simulink model "SiDynoReferenceApplication"  (R2020a)
settings: Solver=ode23tb  StartTime=0.0  StopTime=15000  RelTol=1e-3  EnableMultiTasking=on
model workspace (MAT data in the model file):
  DynOperatingPts = timeseries
  DynOperatingPts.Name = 'Dynamic Operating Points'
  DynOperatingPts.DataInfo = tsdata.datametadata
  DynOperatingPts.DataInfo.Interpolation = tsdata.interpolation
  DynOperatingPts.DataInfo.Interpolation.Fhandle : function handle (value not decoded)
  DynOperatingPts.DataInfo.Interpolation.Name = 'linear'
  DynOperatingPts.TimeInfo = tsdata.timemetadata
  DynOperatingPts.TimeInfo.Length = 1281
  DynOperatingPts.TimeInfo.DuplicateTimes = 0
  DynOperatingPts.TimeInfo.Time_ = [0 0.001 7.75860549558 7.75960549558 8.75958684985 8.76058684985 10.7615495584 10.7625495584 11.7625309127 11.7635309127 13.7644936212 13.7654936212 ... (1281 elements, 1281x1)]
  DynOperatingPts.TimeInfo.Initialized = 1
  DynOperatingPts.QualityInfo = tsdata.qualmetadata
  DynOperatingPts.Data_ = [0 750 750 750 750 750 750 750 750 750 750 750 ... (2562 elements, 1281x2)]
  MaxTurboSpd = 232000
  SteadyEngSpdCmdPts = [750 750 750 750 750 750 750 750 750 750 750 750 ... (225 elements, 15x15)]
  SteadyStateWaitLimit = 100
  SteadyTrqCmdPts = [15 30.3571428571 45.7142857143 61.0714285714 76.4285714286 91.7857142857 107.142857143 122.5 137.857142857 153.214285714 168.571428571 183.928571429 ... (225 elements, 15x15)]
undefined symbols (not defined in the file or in its folder): DynoResultsBlock, GenerateMappedEngineCalibrations, InjPw, RecalibrateSIController, ThrPosPctCmd, WgAreaPctCmd
libraries: autolibutils x2, simulink x2, autolibpowerinfoutils x1
(part 1 of 2)
settings Model: ModifiedByFormat=The MathWorks, Inc.  SimulationMode=accelerator  PauseTimes=4395  NumberOfSteps=1000  SnapshotBufferSize=20  SnapshotInterval=1000  OrderedModelArguments=off  Creator=The MathWorks, Inc.  LastModifiedBy=The MathWorks, Inc.
settings SolverCC: DecoupledContinuousIntegration=on  MinimalZcImpactIntegration=on
settings DataIOCC: SaveOutput=off  SignalLogging=off  DSMLogging=off  SaveTime=off  ReturnWorkspaceOutputs=off
settings OptimizationCC: SimCompilerOptimization=on
settings DebuggingCC: UnderspecifiedInitializationDetection=Classic  MergeDetectMultiDrivingBlocksExec=none  PregeneratedLibrarySubsystemCodeDiagnostic=none  ArithmeticOperatorsInVariantConditions=warning
settings ModelReferenceCC: UpdateModelReferenceTargets=IfOutOfDate  ModelReferenceMinAlgLoopOccurrences=on  PropagateSignalLabelsOutOfModel=off
settings SFSimCC: SimUseLocalCustomCode=off
settings RTWCC: RTWUseLocalCustomCode=off  BuildConfiguration=Faster Runs  RTWCompilerOptimization=on
settings CodeAppCC: StateflowObjectComments=on
settings GRTTargetCC: TargetLangStandard=C89/C90 (ANSI)
settings ConfigComp: CovMetricSettings=dsw  CovHtmlReporting=on  CovSaveCumulativeToWorkspaceVar=on  CovSaveSingleToWorkspaceVar=on  CovShowResultsExplorer=off  CovExternalEMLEnable=off

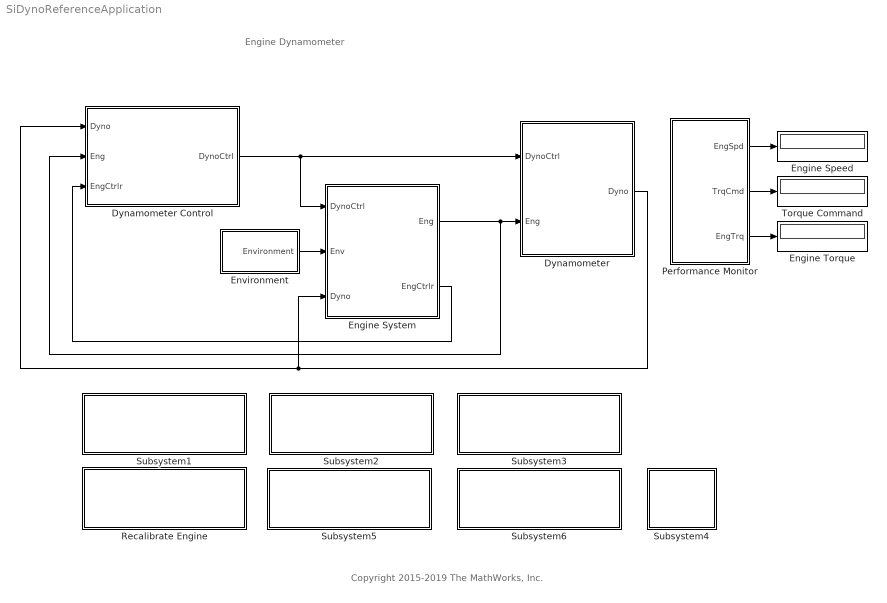
== system SiDynoReferenceApplication ==
  note: Engine Dynamometer
  note: Copyright 2015-2019 The MathWorks, Inc.
  Dynamometer : Subsystem
  Dynamometer Control : Subsystem  Variant=on  VariantControlMode=Label  LabelModeActiveChoice=CalThrWg
  Engine Speed : Display
      settings: Decimation=100
  Engine System : Subsystem
      mask Display:
      | TaggedBlk = find_system(gcb, 'LookUnderMasks', 'All', 'Tag', 'MappedEngCalByMBC');
      | ImageName = which('mbc_app_24.png');
      | 
      | if ~isempty(TaggedBlk)
      |     if ~isempty(ImageName)
      |         IconImg = imread(ImageName,'png');
      |         MaskImg = 256*ones(150, 150,3);
      |         MaskImg = uint8(MaskImg);
      |         Xstart = 125;
      |         Ystart = 0;
      |         MaskImg((1:size(IconImg, 1))+Ystart, (1:size(IconImg, 2))+Xstart, 1:3) = IconImg;
      |         image(MaskImg);
      |     end
      |     disp('Mapped Engine\n Calibrated by\nMBC Toolbox')
      | end
  Engine Torque : Display
      settings: Decimation=100
  Environment : Subsystem
  Performance Monitor : Subsystem  StartFcn=DynoResultsBlock(gcb, 'StartFcn');  StopFcn=DynoResultsBlock(gcb, 'StopFcn');  mask(Performance Monitor){SteadyWsVarName=SteadyDynoSimOut, XVarPopup=Engine speed (rpm), YVarPopup=Torque command (N*m), ZVarPopup=Measured engine torque (N*m), DynWsVarName=DynamicDynoSimOut, DispAtEndCheckbox=on, UseSdiViewCheckbox=on, SdiRunName=Dynamometer Results, SdiViewFileName=DynoSDI_config.mldatx, ShowWaitbarCheckbox=on}
      mask prompts: SteadyWsVarName "Steady state "To Workspace" variable name:"; XVarPopup "X axis variable:"; YVarPopup "Y axis variable:"; ZVarPopup "Z axis variable:"; DynWsVarName "Dynamic "To Workspace" variable name:"; DispAtEndCheckbox "Display results at end of simulation"; UseSdiViewCheckbox "Open Simulation Data Inspector view"; SdiRunName "Simulation Data Inspector run name:"; SdiViewFileName "Simulation Data Inspector view file name:"; ShowWaitbarCheckbox "Show wait bar"
      mask init:
      | DynoResultsBlock(gcb, 'Initialization');
      mask Help: helpview([docroot,'/toolbox/autoblks/helptargets.map'], 'siengine_dyno_refapp')
      mask TypeOptions XVarPopup: Air-fuel ratio | BSFC (g/(kW*hr)) | Compressor outlet temperature (C) | Compressor pressure ratio | EGR cooler outlet temperature (C) | EGR mass flow rate (g/s) | EGR percent | EGR valve area percent | EGR valve area percent command | Engine speed (rpm) | Engine speed command (rpm) | Estimated intake port mass flow rate (g/s) | Exhaust cam phase (degCrkRet) | Exhaust cam phase command (degCrkRet) | Exhaust manifold temperature (C) | Fuel mass flow rate (g/s) | Idle speed control torque command (N*m) | Injection pulse width (ms) | Intake cam phase (degCrkAdv) | Intake cam phase command (degCrkAdv) | Intake manifold pressure (kPa) | Intake manifold temperature (C) | Intake port mass flow rate (g/s) | Intercooler outlet temperature (C) | Load command | Measured engine torque (N*m) | Normalized air charge | Percent complete | Spark advance (degCrkAdv) | Steady state flag | Tailpipe CO emissions (g/s) | Tailpipe CO2 emissions (g/s) | Tailpipe HC emissions (g/s) | Tailpipe NOx emissions (g/s) | Throttle position percent | Throttle position percent command | Time (s) | Torque command (N*m) | Turbine outlet temperature (C) | Turbine pressure ratio | Turbocharger rack position | Turbocharger rack position command | Turbocharger shaft speed (rpm) | Wastegate area percent | Wastegate area percent command
      mask TypeOptions YVarPopup: None | Air-fuel ratio | BSFC (g/(kW*hr)) | Compressor outlet temperature (C) | Compressor pressure ratio | EGR cooler outlet temperature (C) | EGR mass flow rate (g/s) | EGR percent | EGR valve area percent | EGR valve area percent command | Engine speed (rpm) | Engine speed command (rpm) | Estimated intake port mass flow rate (g/s) | Exhaust cam phase (degCrkRet) | Exhaust cam phase command (degCrkRet) | Exhaust manifold temperature (C) | Fuel mass flow rate (g/s) | Idle speed control torque command (N*m) | Injection pulse width (ms) | Intake cam phase (degCrkAdv) | Intake cam phase command (degCrkAdv) | Intake manifold pressure (kPa) | Intake manifold temperature (C) | Intake port mass flow rate (g/s) | Intercooler outlet temperature (C) | Load command | Measured engine torque (N*m) | Normalized air charge | Percent complete | Spark advance (degCrkAdv) | Steady state flag | Tailpipe CO emissions (g/s) | Tailpipe CO2 emissions (g/s) | Tailpipe HC emissions (g/s) | Tailpipe NOx emissions (g/s) | Throttle position percent | Throttle position percent command | Time (s) | Torque command (N*m) | Turbine outlet temperature (C) | Turbine pressure ratio | Turbocharger rack position | Turbocharger rack position command | Turbocharger shaft speed (rpm) | Wastegate area percent | Wastegate area percent command
      mask TypeOptions ZVarPopup: None | Air-fuel ratio | BSFC (g/(kW*hr)) | Compressor outlet temperature (C) | Compressor pressure ratio | EGR cooler outlet temperature (C) | EGR mass flow rate (g/s) | EGR percent | EGR valve area percent | EGR valve area percent command | Engine speed (rpm) | Engine speed command (rpm) | Estimated intake port mass flow rate (g/s) | Exhaust cam phase (degCrkRet) | Exhaust cam phase command (degCrkRet) | Exhaust manifold temperature (C) | Fuel mass flow rate (g/s) | Idle speed control torque command (N*m) | Injection pulse width (ms) | Intake cam phase (degCrkAdv) | Intake cam phase command (degCrkAdv) | Intake manifold pressure (kPa) | Intake manifold temperature (C) | Intake port mass flow rate (g/s) | Intercooler outlet temperature (C) | Load command | Measured engine torque (N*m) | Normalized air charge | Percent complete | Spark advance (degCrkAdv) | Steady state flag | Tailpipe CO emissions (g/s) | Tailpipe CO2 emissions (g/s) | Tailpipe HC emissions (g/s) | Tailpipe NOx emissions (g/s) | Throttle position percent | Throttle position percent command | Time (s) | Torque command (N*m) | Turbine outlet temperature (C) | Turbine pressure ratio | Turbocharger rack position | Turbocharger rack position command | Turbocharger shaft speed (rpm) | Wastegate area percent | Wastegate area percent command
      mask DialogControl SteadyStateGroup Prompt: Steady state
      mask DialogControl SteadyDesc Prompt: Plot steady-state simulation results. Data is logged when an operating point reaches steady state. Once all operating points simulate, the dynamometer outputs data to base workspace. Plot the logged data as a function of 1 or 2 variables. Specify 'None' for the Z axis variable to create a 2D plot. Specify X, Y, and Z variable names to create a surface plot.
      mask DialogControl PlotSteadyButton Prompt: Plot Steady State Results
      mask DialogControl PlotSteadyButton Callback: DynoResultsBlock(gcb, 'PlotSteadyButtonCallback');
      mask DialogControl DynamicGroup Prompt: Dynamic
      mask DialogControl DynamicDesc Prompt: Plot dynamic results using Simulation Data Inspector.
      mask DialogControl PlotDynamicButton Prompt: Plot Dynamic Results
      mask DialogControl PlotDynamicButton Callback: DynoResultsBlock(gcb, 'PlotDynamicButtonCallback');
      mask DialogControl WaitbarGroup Prompt: Wait bar
  Recalibrate Engine : Subsystem  mask{EngReszSpecType=Power, EngReszMaxPwrDesIn=115.0917, EngReszDispDesIn=1.5, EngReszMaxPwrDes=115.0917, EngReszNumCylDes=4, EngReszMaxPwr=115.0917, EngReszNumCyl=4, EngReszDisp=1.5, EngReszIdleSpd=750, EngReszMaxTqSpd=2571, EngReszMaxTq=230.6, EngReszBestFuelPwr=41.1, EngReszBestFuelSpd=2571, EngReszBestFuelTq=152.7, EngReszBestFuelBSFC=225.9, EngReszSpdMaxPwr=5000, EngReszTqMaxPwr=219.8, EngReszThrDiam=50, EngReszIntkManVol=2.86, EngReszExhManVol=1.6, EngReszCompOutVol=2.6, EngReszMaxTurboSpd=232000, EngReszTurboRotInert=0.016, EngReszInjSlp=6.45}
      mask prompts: EngReszSpecType "Power or displacement"; EngReszMaxPwrDesIn "Desired maximum power [kW]:"; EngReszDispDesIn "Desired displacement [L]:"; EngReszMaxPwrDes "Desired maximum power [kW]:"; EngReszNumCylDes "Desired number of cylinders:"; EngReszMaxPwr "Maximum power [kW]:"; EngReszNumCyl "Number of cylinders:"; EngReszDisp "Engine displacement [L]:"; EngReszIdleSpd "Idle speed [rpm]:"; EngReszMaxTqSpd "Speed for maximum torque [rpm]:"; EngReszMaxTq "Maximum torque [Nm]:"; EngReszBestFuelPwr "Power for best fuel [kW]:"; EngReszBestFuelSpd "Speed for best fuel [rpm]:"; EngReszBestFuelTq "Torque for best fuel [Nm]:"; EngReszBestFuelBSFC "BSFC for best fuel [g/kWh]:"; EngReszSpdMaxPwr "Speed for maximum power [rpm]:"; EngReszTqMaxPwr "Torque for maximum power [Nm]:"; EngReszThrDiam "Throttle bore diameter [mm]:"; EngReszIntkManVol "Intake manifold volume [L]:"; EngReszExhManVol "Exhaust manifold volume [L]:"; EngReszCompOutVol "Compressor out volume [L]:"; EngReszMaxTurboSpd "Maximum turbo speed [rpm]:"; EngReszTurboRotInert "Turbo rotor inertia [kg*m^2]:"; EngReszInjSlp "Fuel injector slope [mg/ms]:"
      mask help: Resize engine plant and re-calibrate engine controller based on desired maximum power level or displacement, and number of cylinders
      settings: OpenFcn=|
      | block=[bdroot '/Recalibrate Engine'];
      | 
      | modelStatus = get_param(bdroot,'SimulationStatus');
      | 
      | if ~bdIsLibrary(bdroot) && strcmp(modelStatus,'stopped')
      |    autoicon('autolibsiengresize',block,'open');
      |    open_system(block,'mask');
      | elseif ~bdIsLibrary(bdroot) && ~strcmp(modelStatus,'stopped')
      | else
      | end
      | 
      | clear modelStatus;
      | clear block;
      mask Help: eval('autoblkshelp(''pt_si_resize'')');
      mask TypeOptions EngReszSpecType: Power | Displacement
      mask Callback EngReszSpecType: autoicon('autolibsiengresize',gcb,'resizebasis');
      mask DialogControl DescGroupVar Prompt: Engine resize and recalibrate tool
      mask DialogControl DescTextVar Prompt: Resize engine plant and re-calibrate engine controller based on desired maximum power level or displacement, and number of cylinders
      mask DialogControl ResizeEngButton Prompt: Resize Engine
      mask DialogControl ResizeEngButton Callback: autoicon('autolibsiengresize',gcb,'resize');
      mask DialogControl CurrEngDesign Prompt: Current Engine Design
      mask Display: disp('Resize Engine and\nRecalibrate Controller')
  Subsystem1 : Subsystem
      settings: OpenFcn=DynamometerStart(gcb, 'SteadyState')
      mask Display: disp('Execute Engine Mapping\nExperiment')
  Subsystem2 : Subsystem
      settings: OpenFcn=DynamometerStart(gcb, 'Dynamic')
      mask Display: disp('Execute Model Predictive\nControl Plant Model Experiment')
  Subsystem3 : Subsystem  StopFcn=RecalibrateSIController(gcb, 'StopFcn')
      settings: OpenFcn=RecalibrateSIController(gcb, 'OpenFcn')
      mask Display: disp('Recalibrate Controller')
  Subsystem4 : Subsystem
      settings: OpenFcn=helpview([docroot,'/toolbox/autoblks/helptargets.map'], 'siengine_dyno_refapp')
      mask Display: disp('Help')
  Subsystem5 : Subsystem  LoadFcn=GenerateMappedEngineCalibrations(gcb, 'CheckMBCLicense');  mask(Create Mapped Engine from Spreadsheet){SpreadsheetFileName=SiEngineData.xlsx, MBCProjectName=EngDataMBCProject.mat, CageFileName=MappedEngCageTbls.cag, MappedEngMdlRefName=SiMappedEngine}
      mask prompts: SpreadsheetFileName "Spreadsheet file:"; MBCProjectName "MBC project name:"; CageFileName "CAGE file name:"; MappedEngMdlRefName "Mapped engine model reference name"
      mask help: Use Model-Based Calibration Toolbox to generate a mapped engine calibration from a data spreadsheet. Apply the calibration to a Powertrain Blockset mapped engine model.
      mask init:
      | GenerateMappedEngineCalibrations(gcb, 'Init');
      settings: OpenFcn=open_system(gcb, 'mask')
      mask Help: helpview([docroot,'/toolbox/autoblks/helptargets.map'], 'siengine_dyno_spreadsheet')
      mask DialogControl MBCHyperlink Prompt: Requires Model-Based Calibration Toolbox
      mask DialogControl MBCHyperlink Callback: helpview([docroot,'/toolbox/autoblks/helptargets.map'], 'siengine_dyno_refapp')
      mask DialogControl Container3 Prompt: Step 1: Generate mapped engine calibration using Model-Based Calibration Toolbox
      mask DialogControl SpreadsheetFileNameSelect Prompt: ...
      mask DialogControl SpreadsheetFileNameSelect Callback: GenerateMappedEngineCalibrations(gcb, 'SpreadsheetFileNameSelect');
      mask DialogControl GenMappedEngCalButton Prompt: Generate mapped engine calibration
      mask DialogControl GenMappedEngCalButton Callback: GenerateMappedEngineCalibrations(gcb, 'GenMappedEngCalButton');
      mask DialogControl Container4 Prompt: Step 2: Apply calibration to mapped engine model
      mask DialogControl ApplyCalMappedEngButton Prompt: Apply calibration to mapped engine model
      mask DialogControl ApplyCalMappedEngButton Callback: GenerateMappedEngineCalibrations(gcb, 'ApplyCalMappedEngButton');
      mask Display: disp('Generate Mapped Engine\nfrom Spreadsheet')
  Subsystem6 : Subsystem  mask(Create Mapped Engine from Spreadsheet){SpreadsheetFileName=SiEngineData.xlsx, MBCProjectName=EngDataMBCProject.mat, CageFileName=MappedEngCageTbls.cag, MappedEngMdlRefName=SiMappedEngine}
      mask prompts: SpreadsheetFileName "Spreadsheet file:"; MBCProjectName "MBC project name:"; CageFileName "CAGE file name:"; MappedEngMdlRefName "Mapped engine model reference name"
      mask help: Use Model-Based Calibration Toolbox to generate a mapped engine calibration from a data spreadsheet. Apply the calibration to a Powertrain Blockset mapped engine model.
      mask init:
      | GenerateMappedEngineCalibrations(gcb, 'Init');
      settings: OpenFcn=[~,~,~,~,~,~,~,~,~,~,~,~,~,~]=FitSiEngineLSTM(bdroot(gcb));
      mask Help: helpview([docroot,'/toolbox/autoblks/helptargets.map'], 'siengine_dyno_spreadsheet')
      mask DialogControl MBCHyperlink Prompt: Requires Model-Based Calibration Toolbox
      mask DialogControl MBCHyperlink Callback: helpview([docroot,'/toolbox/autoblks/helptargets.map'], 'siengine_dyno_refapp')
      mask DialogControl Container3 Prompt: Step 1: Generate mapped engine calibration using Model-Based Calibration Toolbox
      mask DialogControl SpreadsheetFileNameSelect Prompt: ...
      mask DialogControl SpreadsheetFileNameSelect Callback: GenerateMappedEngineCalibrations(gcb, 'SpreadsheetFileNameSelect');
      mask DialogControl GenMappedEngCalButton Prompt: Generate mapped engine calibration
      mask DialogControl GenMappedEngCalButton Callback: GenerateMappedEngineCalibrations(gcb, 'GenMappedEngCalButton');
      mask DialogControl Container4 Prompt: Step 2: Apply calibration to mapped engine model
      mask DialogControl ApplyCalMappedEngButton Prompt: Apply calibration to mapped engine model
      mask DialogControl ApplyCalMappedEngButton Callback: GenerateMappedEngineCalibrations(gcb, 'ApplyCalMappedEngButton');
      mask Display: disp('Generate Deep Learning\nEngine Model ')
  Torque Command : Display
      settings: Decimation=100
  wires:
  Performance Monitor/3(EngTrq) -> Engine Torque/1
  Performance Monitor/2(TrqCmd) -> Torque Command/1
  Performance Monitor/1(EngSpd) -> Engine Speed/1
  Engine System/2(EngCtrlr) -> Dynamometer Control/3(EngCtrlr)
  Dynamometer Control/1(DynoCtrl) -> Dynamometer/1(DynoCtrl), Engine System/1(DynoCtrl)
  Dynamometer/1(Dyno) -> Dynamometer Control/1(Dyno), Engine System/3(Dyno)
  Engine System/1(Eng) -> Dynamometer Control/2(Eng), Dynamometer/2(Eng)
  Environment/1(Environment) -> Engine System/2(Env)

== system SiDynoReferenceApplication/Dynamometer ==
  DynoCtrl : Inport
  Eng : Inport  Port=2
  Bus Creator : BusCreator  Inputs=2
  Bus Selector : BusSelector  OutputSignals=EngPlnt.EngTrq,EngPlnt.EngSpd
  Dynamometer Motor Controller : Subsystem
  Dynamometer Plant : Subsystem
  Dyno : Outport  VectorParamsAs1DForOutWhenUnconnected=off
  tag scope: DynoResults=global
  wires:
  Bus Creator/1 -> Dyno/1, [DynoResults]
  Eng/1 -> Bus Selector/1, Dynamometer Plant/1(Eng), Dynamometer Motor Controller/1(EngPlnt)
  Dynamometer Plant/1(DynoPlnt) -> [DynoPlnt], Dynamometer Motor Controller/3(DynoPlnt)
  Dynamometer Motor Controller/1(DynoMotorCtrl) -> Dynamometer Plant/4(DynoCtrl)
  [DynoPlnt] -> Bus Creator/2  "DynoPlnt"
  [DynoCtrl] -> Bus Creator/1  "DynoCtrl"
  DynoCtrl/1 -> [DynoCtrl], Dynamometer Motor Controller/2(DynoCtrl)
  Bus Selector/1 -> Dynamometer Plant/2(EngTrq)  "<EngTrq>"
  Bus Selector/2 -> Dynamometer Plant/3("EngSpd ")  "<EngSpd>"

== system SiDynoReferenceApplication/Dynamometer Control ==
  Dyno : Inport
  Eng : Inport  Port=2
  EngCtrlr : Inport  Port=3
  Calibrate Throttle and Wastegate : Subsystem  VariantControl=CalThrWg
  Dynamic : Subsystem  VariantControl=Dynamic
  Steady State : Subsystem  VariantControl=SteadyState
  DynoCtrl : Outport  VectorParamsAs1DForOutWhenUnconnected=off

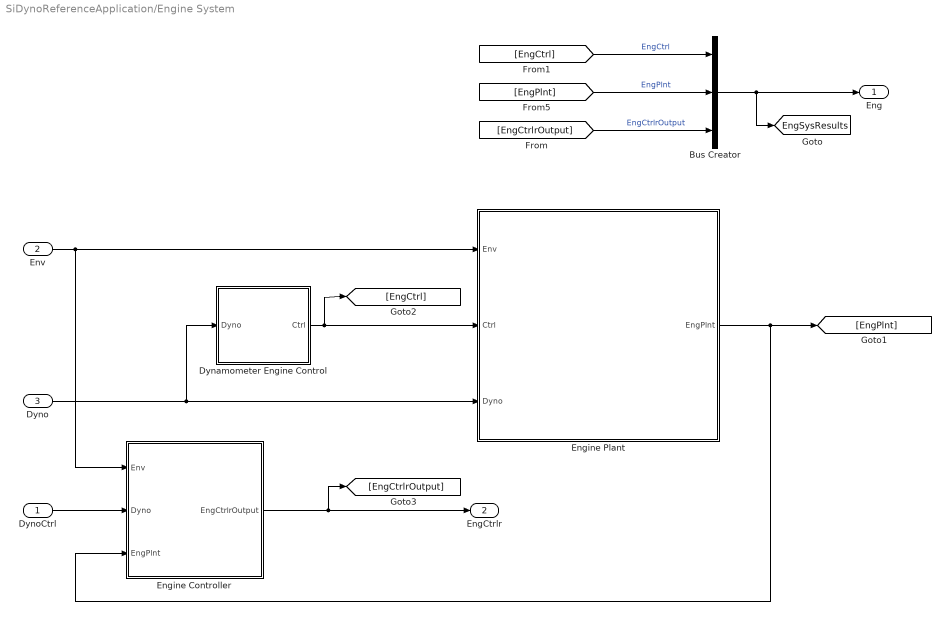
== system SiDynoReferenceApplication/Engine System ==
  DynoCtrl : Inport
  Env : Inport  Port=2
  Dyno : Inport  Port=3
  Bus Creator : BusCreator  Inputs=3
  Dynamometer Engine Control : Subsystem
  Engine Controller : Subsystem
  Engine Plant : Subsystem
  Eng : Outport  VectorParamsAs1DForOutWhenUnconnected=off
  EngCtrlr : Outport  Port=2  VectorParamsAs1DForOutWhenUnconnected=off
  tag scope: EngSysResults=global
  wires:
  Dynamometer Engine Control/1(Ctrl) -> Engine Plant/2(Ctrl), [EngCtrl]
  Dyno/1 -> Dynamometer Engine Control/1(Dyno), Engine Plant/3(Dyno)
  Env/1 -> Engine Controller/1(Env), Engine Plant/1(Env)
  Engine Plant/1(EngPlnt) -> [EngPlnt], Engine Controller/3(EngPlnt)
  Bus Creator/1 -> Eng/1, [EngSysResults]
  [EngPlnt] -> Bus Creator/2  "EngPlnt"
  [EngCtrl] -> Bus Creator/1  "EngCtrl"
  Engine Controller/1(EngCtrlrOutput) -> EngCtrlr/1, [EngCtrlrOutput]
  [EngCtrlrOutput] -> Bus Creator/3  "EngCtrlrOutput"
  DynoCtrl/1 -> Engine Controller/2(Dyno)

== system SiDynoReferenceApplication/Environment ==
  Bus Creator : BusCreator  Inputs=4
  Bus Creator3 : BusCreator  Inputs=3
  Bus Creator4 : BusCreator  Inputs=2
  Bus Creator5 : BusCreator  Inputs=2
  Constant : Constant  Value=1.*ones(4,1)
  Constant1 : Constant  Value=1.*ones(4,1)
  Constant{2..5} (4 alike) : Constant  Value=0
  Constant6 : Constant  Value=300
  Constant7 : Constant  Value=101325
  Environment : Outport  VectorParamsAs1DForOutWhenUnconnected=off
  wires:
  Constant/1 -> Bus Creator5/1  "lam_mu_x"
  Constant1/1 -> Bus Creator5/2  "lam_mu_y"
  Bus Creator5/1 -> Bus Creator4/2  "Ground_mu"
  Bus Creator4/1 -> Bus Creator/3  "Ground"
  Bus Creator3/1 -> Bus Creator/4  "Wind"
  Constant3/1 -> Bus Creator3/1  "wind_x"
  Constant4/1 -> Bus Creator3/2  "wind_y"
  Constant5/1 -> Bus Creator3/3  "wind_z"
  Constant6/1 -> Bus Creator/1  "Temp"
  Constant2/1 -> Bus Creator4/1  "Grade"
  Bus Creator/1 -> Environment/1  "Environment"
  Constant7/1 -> Bus Creator/2  "Baro"

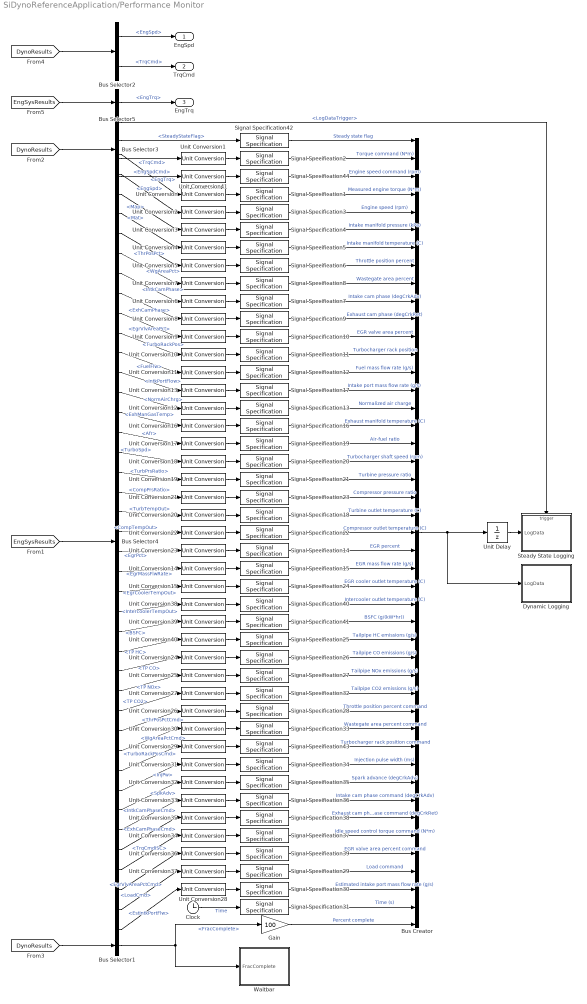
== system SiDynoReferenceApplication/Performance Monitor ==
  Bus Creator : BusCreator  Inputs=45
  Bus Selector1 : BusSelector  OutputSignals=DynoCtrl.DynoCtrl.FracComplete
  Bus Selector2 : BusSelector  OutputSignals=DynoPlnt.EngSpd,DynoCtrl.DynoCtrl.TrqCmd
  Bus Selector3 : BusSelector  OutputSignals=DynoCtrl.DynoCtrl.LogDataTrigger,DynoCtrl.DynoCtrl.SteadyStateFlag,DynoCtrl.DynoCtrl.TrqCmd,DynoCtrl.DynoCtrl.EngSpdCmd
  Bus Selector4 : BusSelector  OutputSignals=EngPlnt.EngTrq,EngPlnt.EngSpd,EngPlnt.Map,EngPlnt.Mat,EngPlnt.ThrPosPct,EngPlnt.WgAreaPct,EngPlnt.IntkCamPhase,EngPlnt.ExhCamPhase,EngPlnt.EgrVlvAreaPct,EngPlnt.TurboRackPos,EngPlnt.FuelFlw,EngPlnt.IntkPortFlow,EngPlnt.NormAirChrg,EngPlnt.ExhManGasTemp,EngPlnt.Afr,EngPlnt.TurboSpd,EngPlnt.TurbPrsRatio,EngPlnt.CompPrsRatio,EngPlnt.TurbTempOut,EngPlnt.CompTempOut,EngPlnt.EgrPct,EngPlnt.EgrMassFlwRate,EngPlnt.EgrCoolerTempOut,EngPlnt.IntercoolerTempOut,EngPlnt.BSFC,EngPlnt.TP HC,EngPlnt.TP CO,EngPlnt.TP NOx,EngPlnt.TP CO2,EngCtrl.ThrPosPctCmd,EngCtrl.WgAreaPctCmd,EngCtrl.TurboRackPosCmd,EngCtrl.InjPw,EngCtrl.SpkAdv,EngCtrl.IntkCamPhaseCmd,EngCtrl.ExhCamPhaseCmd,EngCtrl.TrqCmdISC,EngCtrl.EgrVlvAreaPctCmd,EngCtrl.LoadCmd,EngCtrl.EstIntkPortFlw
  Bus Selector5 : BusSelector  OutputSignals=EngPlnt.EngTrq
  Clock : Clock
  Dynamic Logging : Subsystem
  Gain : Gain  Gain=100
  Signal Specification1 : SignalSpecification  Unit=N*m
  Signal Specification{6,8,10,14,28,33,39} (7 alike) : SignalSpecification  Unit=%
  Signal Specification{11,13,19,21,23,29,42..43} (8 alike) : SignalSpecification  Unit=1
  Signal Specification{12,15,17,25..27,30,32} (8 alike) : SignalSpecification  Unit=g/s
  Signal Specification{5,16,18,22,24,40} (6 alike) : SignalSpecification  Unit=°C
  Signal Specification2 : SignalSpecification  Unit=N*m
  Signal Specification20 : SignalSpecification  Unit=rpm
  Signal Specification3 : SignalSpecification  Unit=rpm
  Signal Specification31 : SignalSpecification  Unit=s
  Signal Specification34 : SignalSpecification  Unit=ms
  Signal Specification{7,9,35..36,38} (5 alike) : SignalSpecification  Unit=deg
  Signal Specification37 : SignalSpecification  Unit=N*m
  Signal Specification4 : SignalSpecification  Unit=kPa
  Signal Specification41 : SignalSpecification  Unit=g/(kW*hr)
  Signal Specification44 : SignalSpecification  Unit=rpm
  Steady State Logging : Subsystem
  Unit Conversion{,1..41} (42 alike) : UnitConversion
  Unit Delay : UnitDelay  SampleTime=-1  HasFrameUpgradeWarning=on
  Waitbar : Subsystem  StartFcn=""
  EngSpd : Outport  VectorParamsAs1DForOutWhenUnconnected=off
  TrqCmd : Outport  Port=2  VectorParamsAs1DForOutWhenUnconnected=off
  EngTrq : Outport  Port=3  VectorParamsAs1DForOutWhenUnconnected=off
  wires:
  Gain/1 -> Bus Creator/45  "Percent complete"
  Signal Specification9/1 -> Bus Creator/11  "Exhaust cam phase (degCrkRet)"
  Signal Specification8/1 -> Bus Creator/9  "Wastegate area percent"
  Signal Specification7/1 -> Bus Creator/10  "Intake cam phase (degCrkAdv)"
  Signal Specification6/1 -> Bus Creator/8  "Throttle position percent"
  Signal Specification5/1 -> Bus Creator/7  "Intake manifold temperature (C)"
  Signal Specification43/1 -> Bus Creator/35  "Turbocharger rack position command"
  Signal Specification41/1 -> Bus Creator/28  "BSFC (g/(kW*hr))"
  Signal Specification40/1 -> Bus Creator/27  "Intercooler outlet temperature (C)"
  Signal Specification4/1 -> Bus Creator/6  "Intake manifold pressure (kPa)"
  Signal Specification39/1 -> Bus Creator/41  "EGR valve area percent command"
  Signal Specification38/1 -> Bus Creator/39  "Exhaust cam phase command (degCrkRet)"
  Signal Specification37/1 -> Bus Creator/40  "Idle speed control torque command (N*m)"
  Signal Specification36/1 -> Bus Creator/38  "Intake cam phase command (degCrkAdv)"
  Signal Specification35/1 -> Bus Creator/37  "Spark advance (degCrkAdv)"
  Signal Specification34/1 -> Bus Creator/36  "Injection pulse width (ms)"
  Signal Specification33/1 -> Bus Creator/34  "Wastegate area percent command"
  Signal Specification32/1 -> Bus Creator/32  "Tailpipe CO2 emissions (g/s)"
  Signal Specification31/1 -> Bus Creator/44  "Time (s)"
  Signal Specification30/1 -> Bus Creator/43  "Estimated intake port mass flow rate (g/s)"
  Signal Specification3/1 -> Bus Creator/5  "Engine speed (rpm)"
  Signal Specification29/1 -> Bus Creator/42  "Load command"
  Signal Specification28/1 -> Bus Creator/33  "Throttle position percent command"
  Signal Specification27/1 -> Bus Creator/31  "Tailpipe NOx emissions (g/s)"
  Signal Specification26/1 -> Bus Creator/30  "Tailpipe CO emissions (g/s)"
  Signal Specification25/1 -> Bus Creator/29  "Tailpipe HC emissions (g/s)"
  Signal Specification24/1 -> Bus Creator/26  "EGR cooler outlet temperature (C)"
  Signal Specification23/1 -> Bus Creator/21  "Compressor pressure ratio"
  Signal Specification22/1 -> Bus Creator/23  "Compressor outlet temperature (C)"
  Signal Specification21/1 -> Bus Creator/20  "Turbine pressure ratio"
  Signal Specification20/1 -> Bus Creator/19  "Turbocharger shaft speed (rpm)"
  Signal Specification19/1 -> Bus Creator/18  "Air-fuel ratio"
  Signal Specification18/1 -> Bus Creator/22  "Turbine outlet temperature (C)"
  Signal Specification17/1 -> Bus Creator/15  "Intake port mass flow rate (g/s)"
  Signal Specification16/1 -> Bus Creator/17  "Exhaust manifold temperature (C)"
  Signal Specification15/1 -> Bus Creator/25  "EGR mass flow rate (g/s)"
  Signal Specification14/1 -> Bus Creator/24  "EGR percent"
  Signal Specification13/1 -> Bus Creator/16  "Normalized air charge"
  Signal Specification12/1 -> Bus Creator/14  "Fuel mass flow rate (g/s)"
  Signal Specification11/1 -> Bus Creator/13  "Turbocharger rack position"
  Signal Specification10/1 -> Bus Creator/12  "EGR valve area percent"
  Signal Specification1/1 -> Bus Creator/4  "Measured engine torque (N*m)"
  Signal Specification44/1 -> Bus Creator/3  "Engine speed command (rpm)"
  Bus Selector3/4 -> Unit Conversion41/1  "<EngSpdCmd>"
  Unit Conversion41/1 -> Signal Specification44/1
  Signal Specification2/1 -> Bus Creator/2  "Torque command (N*m)"
  Bus Selector5/1 -> EngTrq/1  "<EngTrq>"
  [EngSysResults] -> Bus Selector5/1
  Bus Selector2/2 -> TrqCmd/1  "<TrqCmd>"
  Bus Selector2/1 -> EngSpd/1  "<EngSpd>"
  [DynoResults] -> Bus Selector2/1
  [DynoResults] -> Bus Selector1/1
  Bus Selector1/1 -> Gain/1, Waitbar/1(FracComplete)  "<FracComplete>"
  Signal Specification42/1 -> Bus Creator/1  "Steady state flag"
  Bus Selector4/40 -> Unit Conversion28/1  "<EstIntkPortFlw>"
  Bus Selector4/39 -> Unit Conversion37/1  "<LoadCmd>"
  Bus Selector4/38 -> Unit Conversion36/1  "<EgrVlvAreaPctCmd>"
  Bus Selector4/37 -> Unit Conversion34/1  "<TrqCmdISC>"
  Bus Selector4/36 -> Unit Conversion35/1  "<ExhCamPhaseCmd>"
  Bus Selector4/35 -> Unit Conversion33/1  "<IntkCamPhaseCmd>"
  Bus Selector4/34 -> Unit Conversion32/1  "<SpkAdv>"
  Bus Selector4/33 -> Unit Conversion31/1  "<InjPw>"
  Bus Selector4/31 -> Unit Conversion30/1  "<WgAreaPctCmd>"
  Bus Selector4/30 -> Unit Conversion26/1  "<ThrPosPctCmd>"
  Bus Selector4/29 -> Unit Conversion27/1  "<TP CO2>"
  Bus Selector4/28 -> Unit Conversion25/1  "<TP NOx>"
  Bus Selector4/27 -> Unit Conversion24/1  "<TP CO>"
  Bus Selector4/26 -> Unit Conversion40/1  "<TP HC>"
  Bus Selector4/25 -> Unit Conversion39/1  "<BSFC>"
  Bus Selector4/24 -> Unit Conversion38/1  "<IntercoolerTempOut>"
  Unit Conversion28/1 -> Signal Specification30/1
  Unit Conversion37/1 -> Signal Specification29/1
  Unit Conversion36/1 -> Signal Specification39/1
  Unit Conversion35/1 -> Signal Specification38/1
  Unit Conversion34/1 -> Signal Specification37/1
  Unit Conversion33/1 -> Signal Specification36/1
  Unit Conversion32/1 -> Signal Specification35/1
  Unit Conversion31/1 -> Signal Specification34/1
  Unit Conversion30/1 -> Signal Specification33/1
  Unit Conversion27/1 -> Signal Specification32/1
  Unit Conversion26/1 -> Signal Specification28/1
  Unit Conversion25/1 -> Signal Specification27/1
  Unit Conversion24/1 -> Signal Specification26/1
  Unit Conversion40/1 -> Signal Specification25/1
  Unit Conversion39/1 -> Signal Specification41/1
  Unit Conversion38/1 -> Signal Specification40/1
  Bus Selector4/23 -> Unit Conversion15/1  "<EgrCoolerTempOut>"
  Bus Selector4/22 -> Unit Conversion14/1  "<EgrMassFlwRate>"
  Bus Selector4/21 -> Unit Conversion23/1  "<EgrPct>"
  Bus Selector4/20 -> Unit Conversion22/1  "<CompTempOut>"
  Bus Selector4/19 -> Unit Conversion20/1  "<TurbTempOut>"
  Bus Selector4/18 -> Unit Conversion21/1  "<CompPrsRatio>"
  Bus Selector4/17 -> Unit Conversion19/1  "<TurbPrsRatio>"
  Bus Selector4/16 -> Unit Conversion18/1  "<TurboSpd>"
  Bus Selector4/15 -> Unit Conversion17/1  "<Afr>"
  Bus Selector4/14 -> Unit Conversion16/1  "<ExhManGasTemp>"
  Bus Selector4/13 -> Unit Conversion12/1  "<NormAirChrg>"
  Bus Selector4/12 -> Unit Conversion13/1  "<IntkPortFlow>"
  Unit Conversion15/1 -> Signal Specification24/1
  Unit Conversion14/1 -> Signal Specification15/1
  Unit Conversion23/1 -> Signal Specification14/1
  Unit Conversion22/1 -> Signal Specification22/1
  Unit Conversion21/1 -> Signal Specification23/1
  Unit Conversion20/1 -> Signal Specification18/1
  Unit Conversion19/1 -> Signal Specification21/1
  Unit Conversion18/1 -> Signal Specification20/1
  Unit Conversion17/1 -> Signal Specification19/1
  Unit Conversion16/1 -> Signal Specification16/1
  Unit Conversion13/1 -> Signal Specification17/1
  Unit Conversion12/1 -> Signal Specification13/1
  Bus Selector4/11 -> Unit Conversion11/1  "<FuelFlw>"
  Bus Selector4/10 -> Unit Conversion10/1  "<TurboRackPos>"
  Bus Selector4/9 -> Unit Conversion9/1  "<EgrVlvAreaPct>"
  Bus Selector4/8 -> Unit Conversion8/1  "<ExhCamPhase>"
  Bus Selector4/7 -> Unit Conversion6/1  "<IntkCamPhase>"
  Bus Selector4/6 -> Unit Conversion7/1  "<WgAreaPct>"
  Unit Conversion11/1 -> Signal Specification12/1
  Unit Conversion10/1 -> Signal Specification11/1
  Unit Conversion9/1 -> Signal Specification10/1
  Unit Conversion8/1 -> Signal Specification9/1
  Unit Conversion7/1 -> Signal Specification8/1
  Unit Conversion6/1 -> Signal Specification7/1
  Bus Selector4/5 -> Unit Conversion5/1  "<ThrPosPct>"
  Unit Conversion5/1 -> Signal Specification6/1
  Bus Selector4/4 -> Unit Conversion4/1  "<Mat>"
  Unit Conversion4/1 -> Signal Specification5/1
  Unit Conversion3/1 -> Signal Specification4/1
  Unit Conversion2/1 -> Signal Specification3/1
  Unit Conversion1/1 -> Signal Specification2/1
  Unit Conversion/1 -> Signal Specification1/1
  Clock/1 -> Signal Specification31/1  "Time"
  Bus Selector3/2 -> Signal Specification42/1  "<SteadyStateFlag>"
  Bus Selector3/3 -> Unit Conversion1/1  "<TrqCmd>"
  Bus Selector3/1 -> Steady State Logging/Trigger  "<LogDataTrigger>"
  [EngSysResults] -> Bus Selector4/1
  [DynoResults] -> Bus Selector3/1
  Bus Selector4/1 -> Unit Conversion/1  "<EngTrq>"
  Bus Selector4/2 -> Unit Conversion2/1  "<EngSpd>"
  Bus Selector4/3 -> Unit Conversion3/1  "<Map>"
  Bus Creator/1 -> Unit Delay/1, Dynamic Logging/1(LogData)
  Unit Delay/1 -> Steady State Logging/1(LogData)
  Unit Conversion29/1 -> Signal Specification43/1
  Bus Selector4/32 -> Unit Conversion29/1  "<TurboRackPosCmd>"

== system SiDynoReferenceApplication/Recalibrate Engine ==

== system SiDynoReferenceApplication/Subsystem1 ==

== system SiDynoReferenceApplication/Subsystem2 ==

== system SiDynoReferenceApplication/Subsystem3 ==

== system SiDynoReferenceApplication/Subsystem4 ==

== system SiDynoReferenceApplication/Subsystem5 ==

== system SiDynoReferenceApplication/Subsystem6 ==

== system SiDynoReferenceApplication/Dynamometer/Dynamometer Motor Controller ==
  EngPlnt : Inport
  DynoCtrl : Inport  Port=2
  DynoPlnt : Inport  Port=3
  Bus Creator : BusCreator  Inputs=2
  Bus Selector : BusSelector  OutputSignals=DynoCtrl.EngSpdCmd,DynoCtrl.FanFlwSpdCmd
  Terminator : Terminator
  Terminator1 : Terminator
  DynoMotorCtrl : Outport  VectorParamsAs1DForOutWhenUnconnected=off
  wires:
  DynoCtrl/1 -> Bus Selector/1
  EngPlnt/1 -> Terminator/1
  DynoPlnt/1 -> Terminator1/1
  Bus Selector/1 -> Bus Creator/1  "<EngSpdCmd>"
  Bus Creator/1 -> DynoMotorCtrl/1
  Bus Selector/2 -> Bus Creator/2  "<FanFlwSpdCmd>"

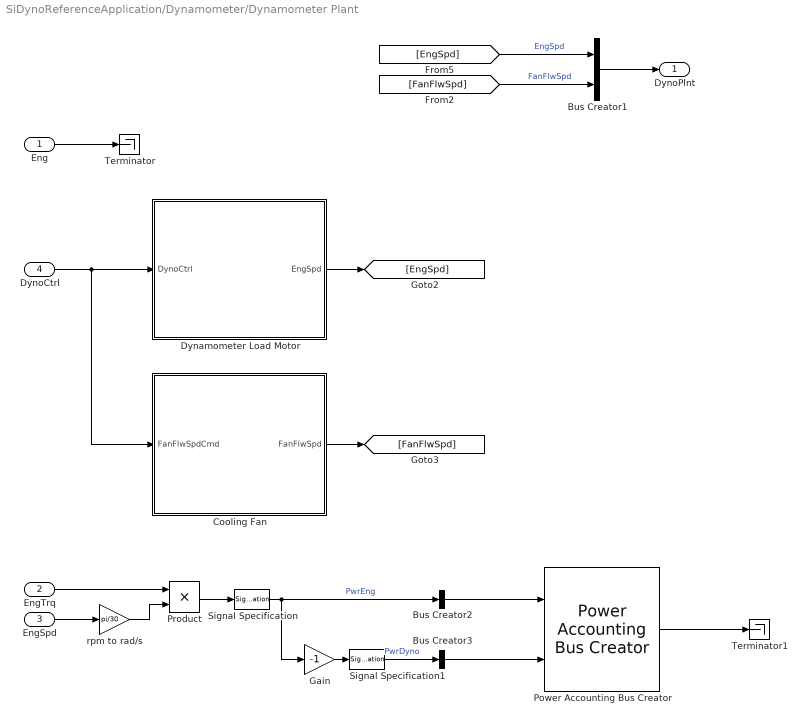
== system SiDynoReferenceApplication/Dynamometer/Dynamometer Plant ==
  Eng : Inport
  EngTrq : Inport  Port=2
  "EngSpd " : Inport  Port=3
  DynoCtrl : Inport  Port=4
  Bus Creator1 : BusCreator  Inputs=2
  Bus Creator2 : BusCreator  Inputs=1
  Bus Creator3 : BusCreator  Inputs=1
  Cooling Fan : Subsystem
  Dynamometer Load Motor : Subsystem
  Gain : Gain  Gain=-1
  Power Accounting Bus Creator : autolibpowerinfoutils/Power Accounting Bus Creator  AssctBlkSelPopup=Parent  RefBlkName='libraryname/blkname'  PwrTrnsfrdCheckBox=on  PwrNotTrnsfrdCheckBox=on  PwrStoredCheckBox=off  aMode=aMode
      settings: SourceProductBaseCode=PW,MT,VE,VP
  Product : Product
  Signal Specification : SignalSpecification  Unit=W
  Signal Specification1 : SignalSpecification  Unit=W
  Terminator : Terminator
  Terminator1 : Terminator
  rpm to rad/s : Gain  Gain=pi/30
  DynoPlnt : Outport  VectorParamsAs1DForOutWhenUnconnected=off
  wires:
  Cooling Fan/1(FanFlwSpd) -> [FanFlwSpd]
  Dynamometer Load Motor/1(EngSpd) -> [EngSpd]
  Bus Creator1/1 -> DynoPlnt/1
  [EngSpd] -> Bus Creator1/1  "EngSpd"
  [FanFlwSpd] -> Bus Creator1/2  "FanFlwSpd"
  DynoCtrl/1 -> Cooling Fan/1(FanFlwSpdCmd), Dynamometer Load Motor/1(DynoCtrl)
  Eng/1 -> Terminator/1
  Bus Creator2/1 -> Power Accounting Bus Creator/1
  Signal Specification/1 -> Gain/1, Bus Creator2/1  "PwrEng"
  Bus Creator3/1 -> Power Accounting Bus Creator/2
  Power Accounting Bus Creator/1 -> Terminator1/1
  Gain/1 -> Signal Specification1/1
  Product/1 -> Signal Specification/1
  Signal Specification1/1 -> Bus Creator3/1  "PwrDyno"
  EngTrq/1 -> Product/1
  "EngSpd "/1 -> rpm to rad/s/1
  rpm to rad/s/1 -> Product/2

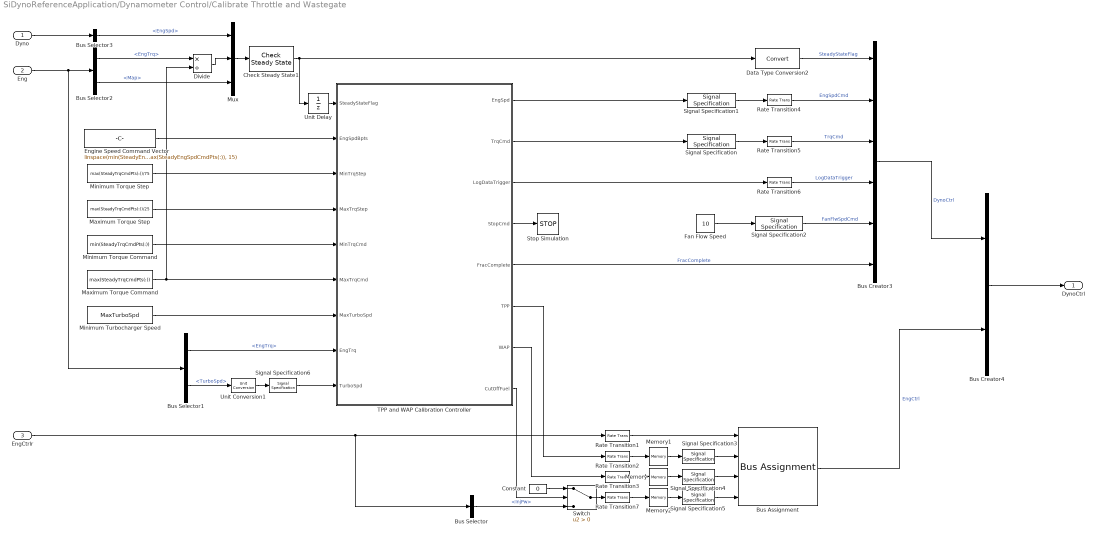
== system SiDynoReferenceApplication/Dynamometer Control/Calibrate Throttle and Wastegate ==
  Dyno : Inport
  Eng : Inport  Port=2
  EngCtrlr : Inport  Port=3
  Bus Assignment : BusAssignment  AssignedSignals=ThrPosPctCmd,WgAreaPctCmd,InjPw
  Bus Creator3 : BusCreator  Inputs=6
  Bus Creator4 : BusCreator  Inputs=2
  Bus Selector : BusSelector  OutputSignals=InjPw
  Bus Selector1 : BusSelector  OutputSignals=EngPlnt.EngTrq,EngPlnt.TurboSpd
  Bus Selector2 : BusSelector  OutputSignals=EngPlnt.EngTrq,EngPlnt.Map
  Bus Selector3 : BusSelector  OutputSignals=DynoPlnt.EngSpd
  Check Steady State1 : autolibutils/Check Steady State  N=4  F=50  Ts=0.2  SteadyThresh=[0.1; 0.002; 500]  HoldTime=0.5  aMode=aMode
      settings: SourceProductBaseCode=PW,MT,VE,VP
  Constant : Constant  Value=0
  Data Type Conversion2 : DataTypeConversion
  Divide : Product  Inputs=*/
  Engine Speed Command Vector : Constant  Value=linspace(min(SteadyEngSpdCmdPts(:)), max(SteadyEngSpdCmdPts(:)), 15)
  Fan Flow Speed : Constant  Value=10
  Maximum Torque Command : Constant  Value=max(SteadyTrqCmdPts(:))
  Maximum Torque Step : Constant  Value=max(SteadyTrqCmdPts(:))/25
  Memory : Memory  InitialCondition=100
  Memory1 : Memory
  Memory2 : Memory  InitialCondition=100
  Minimum Torque Command : Constant  Value=min(SteadyTrqCmdPts(:))
  Minimum Torque Step : Constant  Value=max(SteadyTrqCmdPts(:))/75
  Minimum Turbocharger Speed : Constant  Value=MaxTurboSpd
  Mux : Mux  Inputs=3
  Rate Transition{1..3,7} (4 alike) : RateTransition  Deterministic=off  OutPortSampleTimeOpt=Inherit
  Rate Transition4 : RateTransition  Deterministic=off
  Rate Transition5 : RateTransition  Deterministic=off
  Rate Transition6 : RateTransition  Deterministic=off
  Signal Specification : SignalSpecification  Unit=N*m
  Signal Specification1 : SignalSpecification  Unit=rpm
  Signal Specification2 : SignalSpecification  Unit=N*m
  Signal Specification3 : SignalSpecification  Unit=%
  Signal Specification4 : SignalSpecification  Unit=%
  Signal Specification5 : SignalSpecification  Unit=ms
  Signal Specification6 : SignalSpecification  Unit=rpm
  Stop Simulation : Stop
  Switch : Switch  Criteria=u2 > Threshold
  TPP and WAP Calibration Controller : Stateflow chart  TreatAsAtomicUnit=on
  Unit Conversion1 : UnitConversion
  Unit Delay : UnitDelay  SampleTime=-1  HasFrameUpgradeWarning=on
  DynoCtrl : Outport  VectorParamsAs1DForOutWhenUnconnected=off
  wires:
  Divide/1 -> Mux/2
  Bus Selector3/1 -> Mux/1  "<EngSpd>"
  Bus Selector2/1 -> Divide/1  "<EngTrq>"
  TPP and WAP Calibration Controller/2(TrqCmd) -> Signal Specification/1
  Bus Selector2/2 -> Mux/3  "<Map>"
  TPP and WAP Calibration Controller/7(WAP) -> Rate Transition3/1
  TPP and WAP Calibration Controller/6(TPP) -> Rate Transition2/1
  Bus Creator3/1 -> Bus Creator4/1  "DynoCtrl"
  Bus Creator4/1 -> DynoCtrl/1
  Mux/1 -> Check Steady State1/1
  Data Type Conversion2/1 -> Bus Creator3/1  "SteadyStateFlag"
  Rate Transition6/1 -> Bus Creator3/4  "LogDataTrigger"
  Rate Transition5/1 -> Bus Creator3/3  "TrqCmd"
  Rate Transition4/1 -> Bus Creator3/2  "EngSpdCmd"
  Fan Flow Speed/1 -> Signal Specification2/1
  Maximum Torque Step/1 -> TPP and WAP Calibration Controller/4(MaxTrqStep)
  Engine Speed Command Vector/1 -> TPP and WAP Calibration Controller/2(EngSpdBpts)
  TPP and WAP Calibration Controller/4(StopCmd) -> Stop Simulation/1
  Dyno/1 -> Bus Selector3/1
  Eng/1 -> Bus Selector1/1, Bus Selector2/1
  Rate Transition3/1 -> Memory/1
  Rate Transition2/1 -> Memory1/1
  Bus Selector1/1 -> TPP and WAP Calibration Controller/8(EngTrq)  "<EngTrq>"
  Bus Selector1/2 -> Unit Conversion1/1  "<TurboSpd>"
  Signal Specification/1 -> Rate Transition5/1
  Signal Specification1/1 -> Rate Transition4/1
  TPP and WAP Calibration Controller/1(EngSpd) -> Signal Specification1/1
  Signal Specification2/1 -> Bus Creator3/5  "FanFlwSpdCmd"
  TPP and WAP Calibration Controller/5(FracComplete) -> Bus Creator3/6  "FracComplete"
  EngCtrlr/1 -> Rate Transition1/1, Bus Selector/1
  Memory/1 -> Signal Specification4/1
  Memory1/1 -> Signal Specification3/1
  Bus Assignment/1 -> Bus Creator4/2  "EngCtrl"
  Signal Specification3/1 -> Bus Assignment/2
  Signal Specification4/1 -> Bus Assignment/3
  Rate Transition1/1 -> Bus Assignment/1
  Minimum Torque Step/1 -> TPP and WAP Calibration Controller/3(MinTrqStep)
  Minimum Torque Command/1 -> TPP and WAP Calibration Controller/5(MinTrqCmd)
  Maximum Torque Command/1 -> Divide/2, TPP and WAP Calibration Controller/6(MaxTrqCmd)
  Check Steady State1/1 -> Unit Delay/1, Data Type Conversion2/1
  TPP and WAP Calibration Controller/3(LogDataTrigger) -> Rate Transition6/1
  Minimum Turbocharger Speed/1 -> TPP and WAP Calibration Controller/7(MaxTurboSpd)
  Unit Conversion1/1 -> Signal Specification6/1
  Signal Specification6/1 -> TPP and WAP Calibration Controller/9(TurboSpd)
  Memory2/1 -> Signal Specification5/1
  Rate Transition7/1 -> Memory2/1
  Signal Specification5/1 -> Bus Assignment/4
  Switch/1 -> Rate Transition7/1
  TPP and WAP Calibration Controller/8(CutOffFuel) -> Switch/2
  Constant/1 -> Switch/1
  Bus Selector/1 -> Switch/3  "<InjPw>"
  Unit Delay/1 -> TPP and WAP Calibration Controller/1(SteadyStateFlag)

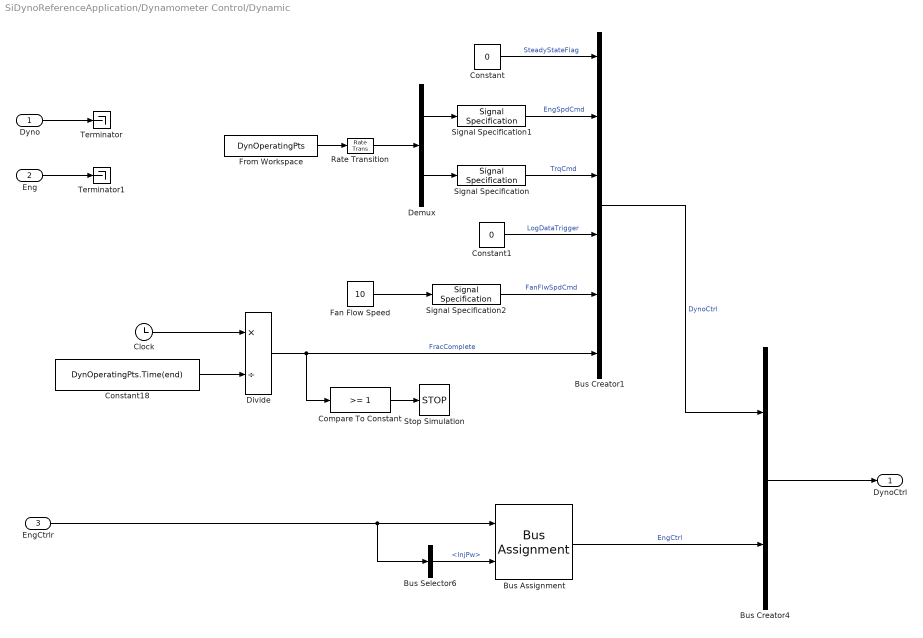
== system SiDynoReferenceApplication/Dynamometer Control/Dynamic ==
  Dyno : Inport
  Eng : Inport  Port=2
  EngCtrlr : Inport  Port=3
  Bus Assignment : BusAssignment  AssignedSignals=InjPw
  Bus Creator1 : BusCreator  Inputs=6
  Bus Creator4 : BusCreator  Inputs=2
  Bus Selector6 : BusSelector  OutputSignals=InjPw
  Clock : Clock
  Compare To Constant : simulink/Logic and Bit Operations/Compare To Constant  relop=>=  const=1  OutDataTypeStr=boolean
  Constant : Constant  Value=0
  Constant1 : Constant  Value=0
  Constant18 : Constant  Value=DynOperatingPts.Time(end)
  Demux : Demux  Outputs=2
  Divide : Product  Inputs=*/
  Fan Flow Speed : Constant  Value=10
  From Workspace : FromWorkspace  VariableName=DynOperatingPts  SampleTime=0.01  ZeroCross=off  OutputAfterFinalValue=Holding final value
  Rate Transition : RateTransition
  Signal Specification : SignalSpecification  Unit=N*m
  Signal Specification1 : SignalSpecification  Unit=rpm
  Signal Specification2 : SignalSpecification  Unit=m/s
  Stop Simulation : Stop
  Terminator : Terminator
  Terminator1 : Terminator
  DynoCtrl : Outport  VectorParamsAs1DForOutWhenUnconnected=off
  wires:
  Bus Creator1/1 -> Bus Creator4/1  "DynoCtrl"
  Bus Creator4/1 -> DynoCtrl/1
  Constant1/1 -> Bus Creator1/4  "LogDataTrigger"
  Constant/1 -> Bus Creator1/1  "SteadyStateFlag"
  Dyno/1 -> Terminator/1
  Demux/1 -> Signal Specification1/1
  Demux/2 -> Signal Specification/1
  Clock/1 -> Divide/1
  Compare To Constant/1 -> Stop Simulation/1
  From Workspace/1 -> Rate Transition/1
  Rate Transition/1 -> Demux/1
  Fan Flow Speed/1 -> Signal Specification2/1
  Signal Specification2/1 -> Bus Creator1/5  "FanFlwSpdCmd"
  Signal Specification1/1 -> Bus Creator1/2  "EngSpdCmd"
  Signal Specification/1 -> Bus Creator1/3  "TrqCmd"
  Divide/1 -> Compare To Constant/1, Bus Creator1/6  "FracComplete"
  Constant18/1 -> Divide/2
  EngCtrlr/1 -> Bus Assignment/1, Bus Selector6/1
  Bus Assignment/1 -> Bus Creator4/2  "EngCtrl"
  Bus Selector6/1 -> Bus Assignment/2  "<InjPw>"
  Eng/1 -> Terminator1/1
